simulink model "task1-Simulink"  (R2015b)
settings: Solver=VariableStepAuto  StartTime=0.0  StopTime=0.2  RelTol=1e-3
values from neighbouring files (symbols this model uses):
  A = [0 0 0 1 0 0;     0 0 0 0 1 0;      0 0 0 0 0 1;     (kt-ko)/J1 kt/(J1*n^2) -kt/J1 (dt-do)/J1 dt/(J1*n^2) -dt/J1;    -kt/(Jmg*n^2) -kt/((n^4)*Jmg) kt/((n^2)*Jmg) -dt/(Jmg*n^2) 1/Jmg*(-Km*Kemf/R-dt/(n^4)) dt/(n^2*Jmg);    kt/Jout kt/((n^2)*Jout) (-kt-kr)/Jout dt/Jout dt/((n^2)*Jout) -(dt+dj)/Jout]    [All Tasks Compiled.m]
  B = [0 0 0 0 Km/(R*Jmg) 0]'    [All Tasks Compiled.m]
  C = eye(6)    [All Tasks Compiled.m]
  D = [0 0 0 0 0 0]'    [All Tasks Compiled.m]
  d = 8/1000    (= 0.008)    [All Tasks Compiled.m]
  J = 60*10^-7    (= 6e-06)    [All Tasks Compiled.m]
  Kemf = 4.555*10^(-3)*60/(2*pi)    (= 0.043497045947)    [All Tasks Compiled.m]
  Km = 43.5*10^-3    (= 0.0435)    [All Tasks Compiled.m]
  L = 0.1    [All Tasks Compiled.m]
  n = sqrt(t2/Mh)    [All Tasks Compiled.m]
  R = 1.45    [All Tasks Compiled.m]
settings Model: Creator=atang  LastModifiedBy=daniella.a
settings DataIOCC: LimitDataPoints=off

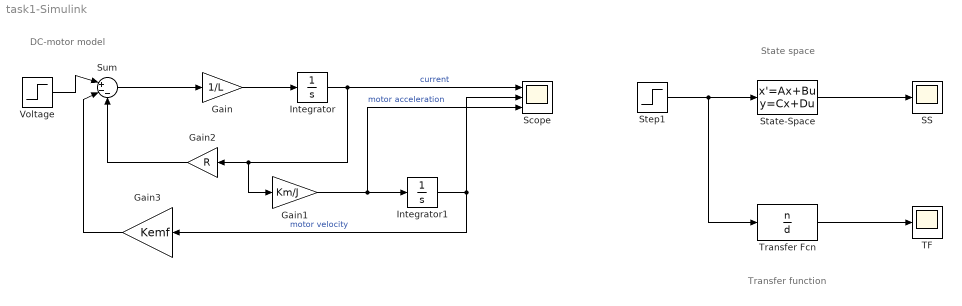
== system task1-Simulink ==
  note: Transfer function
  note: State space
  note: DC-motor model
  Gain : Gain  Gain=1/L
  Gain1 : Gain  Gain=Km/J
  Gain2 : Gain  Gain=R
  Gain3 : Gain  Gain=Kemf
  Integrator : Integrator
  Integrator1 : Integrator
  SS : Scope
  Scope : Scope  NumInputPorts=3
  State-Space : StateSpace  A=A  B=B  C=C  D=D  X0=0
  Step1 : Step  After=24  SampleTime=0
  Sum : Sum  Inputs=|+--
  TF : Scope
  Transfer Fcn : TransferFcn  Numerator=n  Denominator=d
  Voltage : Step  Time=0  After=24  SampleTime=0
  wires:
  Sum/1 -> Gain/1
  Voltage/1 -> Sum/1
  Gain/1 -> Integrator/1
  Integrator/1 -> Scope/1, Gain1/1, Gain2/1  "current"
  Gain2/1 -> Sum/3
  Gain1/1 -> Integrator1/1, Scope/3  "motor acceleration"
  Integrator1/1 -> Gain3/1, Scope/2  "motor velocity"
  Gain3/1 -> Sum/2
  State-Space/1 -> SS/1
  Step1/1 -> Transfer Fcn/1, State-Space/1
  Transfer Fcn/1 -> TF/1
